simulink model "VTOLDynamics"  (R2024b)
settings: Solver=ode23t  StartTime=0.0  StopTime=10.0  FixedStep=0.001  RelTol=1e-3
undefined symbols (not defined in the file): const, contact, env, F, Flap_Activate, iniRoll, initPitch, iniYaw, Light, Limit, MIL, motorctrl, tiltIni, uavParam, uavParams, vIni, xGround, yGround, zGround
libraries: matrix_library x8, slpidlib x4, robotcorelib x4, aerolibasang x2, aerolibwind2 x2, sharedtransform x2, shared6dof x1, aerolibadyn x1, sharedutil x1, Uav_Electrical_lib x1, aerolibatmos2 x1
(part 1 of 3)
settings Model: DataDictionary=VTOLDynamicsData.sldd  Creator=The MathWorks, Inc.  LastModifiedBy=soung
settings DataIOCC: SaveOutput=off  SaveTime=off
settings GRTTargetCC: CombineOutputUpdateFcns=off  MatFileLogging=off

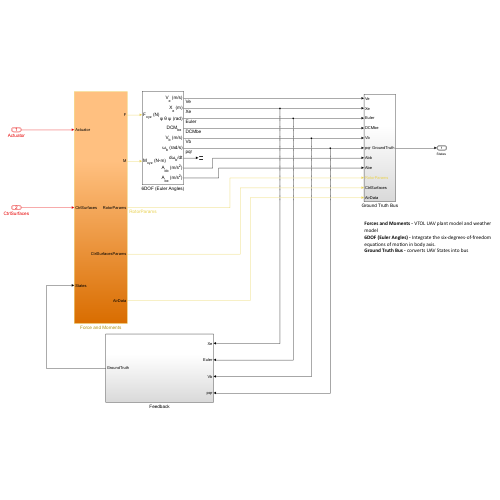
[thumbnail: Simulink's stored preview of the top-level diagram]
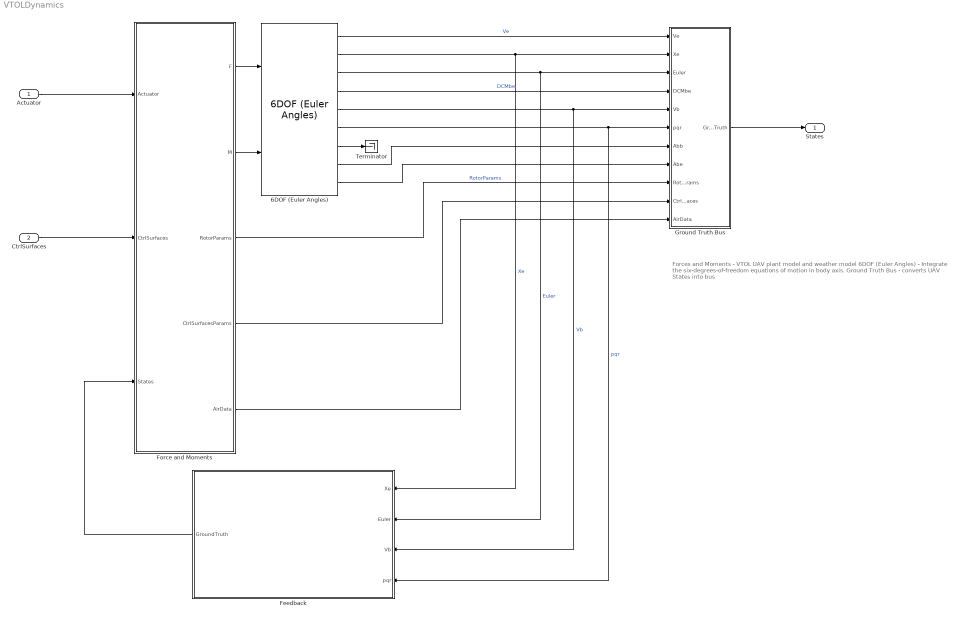
== system VTOLDynamics ==
  note: Forces and Moments - VTOL UAV plant model and weather model
      | 6DOF (Euler Angles) - Integrate the six-degrees-of-freedom equations of motion in body axis.
      | Ground Truth Bus - converts UAV States into bus
  Actuator : Inport  OutDataTypeStr=Bus: RotorCtrlBus  BusOutputAsStruct=on
  CtrlSurfaces : Inport  Port=2  OutDataTypeStr=Bus: FixedWingCtrlBus  BusOutputAsStruct=on
  6DOF (Euler Angles) : shared6dof/6DOF (Euler Angles)  units=Metric (MKS)  mtype=Fixed  rep=Euler Angles  xme_0=[xGround yGround zGround]  Vm_0=[vIni 0 0]  eul_0=[iniRoll initPitch iniYaw]  pm_0=[0 0 0]  mass_0=uavParams.geom.mass  mass_e=0.5  mass_f=2.0  inertia=[uavParams.geom.Ixx 0 0; 0 uavParams.geom.Iyy 0; 0 0 uavParams.geom.Izz]  inertia_e=eye(3)  inertia_f=2*eye(3)  k_quat=1.0  vre_flag=on  abi_flag=on  aMode=0  xme_statename=''  Vm_statename=''  eul_statename=''  quat_statename=''  pm_statename=''  mass_statename=''
  Feedback : Subsystem
  Force and Moments : Subsystem
  Ground Truth Bus : Subsystem
  Terminator : Terminator
  "States " : Outport  OutDataTypeStr=Bus: stateBus  BusOutputAsStruct=on
  wires:
  6DOF (Euler Angles)/4 -> Ground Truth Bus/4(DCMbe)  "DCMbe"
  Actuator/1 -> Force and Moments/1(Actuator)
  6DOF (Euler Angles)/2 -> Feedback/1(Xe), Ground Truth Bus/2(Xe)  "Xe"
  Force and Moments/5(AirData) -> Ground Truth Bus/11(AirData)
  6DOF (Euler Angles)/1 -> Ground Truth Bus/1(Ve)  "Ve"
  Force and Moments/3(RotorParams) -> Ground Truth Bus/9(RotorParams)  "RotorParams"
  6DOF (Euler Angles)/6 -> Ground Truth Bus/6(pqr), Feedback/4(pqr)  "pqr"
  CtrlSurfaces/1 -> Force and Moments/2(CtrlSurfaces)
  6DOF (Euler Angles)/7 -> Terminator/1
  6DOF (Euler Angles)/3 -> Feedback/2(Euler), Ground Truth Bus/3(Euler)  "Euler"
  6DOF (Euler Angles)/5 -> Ground Truth Bus/5(Vb), Feedback/3(Vb)  "Vb"
  Ground Truth Bus/1(GroundTruth) -> "States "/1
  6DOF (Euler Angles)/8 -> Ground Truth Bus/7(Abb)
  6DOF (Euler Angles)/9 -> Ground Truth Bus/8(Abe)
  Force and Moments/1(F) -> 6DOF (Euler Angles)/1
  Force and Moments/2(M) -> 6DOF (Euler Angles)/2
  Force and Moments/4(CtrlSurfacesParams) -> Ground Truth Bus/10(CtrlSurfaces)
  Feedback/1(GroundTruth) -> Force and Moments/3(States)

== system VTOLDynamics/Feedback ==
  Xe : Inport
  Euler : Inport  Port=2
  Vb : Inport  Port=3
  pqr : Inport  Port=4
  Reshape{,1..3} (4 alike) : Reshape  OutputDimensionality=Column vector (2-D)
  Bus Element Out3 : Outport  PortName=GroundTruth  Element=Xe
  Bus Element Out9 : Outport  PortName=GroundTruth  Element=pqr
  Bus Element Out6 : Outport  PortName=GroundTruth  Element=Vb
  Bus Element Out5 : Outport  PortName=GroundTruth  Element=Euler
  wires:
  Vb/1 -> Reshape/1
  Euler/1 -> Reshape1/1
  pqr/1 -> Reshape3/1
  Xe/1 -> Reshape2/1
  Reshape/1 -> Bus Element Out6/1
  Reshape1/1 -> Bus Element Out5/1
  Reshape2/1 -> Bus Element Out3/1
  Reshape3/1 -> Bus Element Out9/1

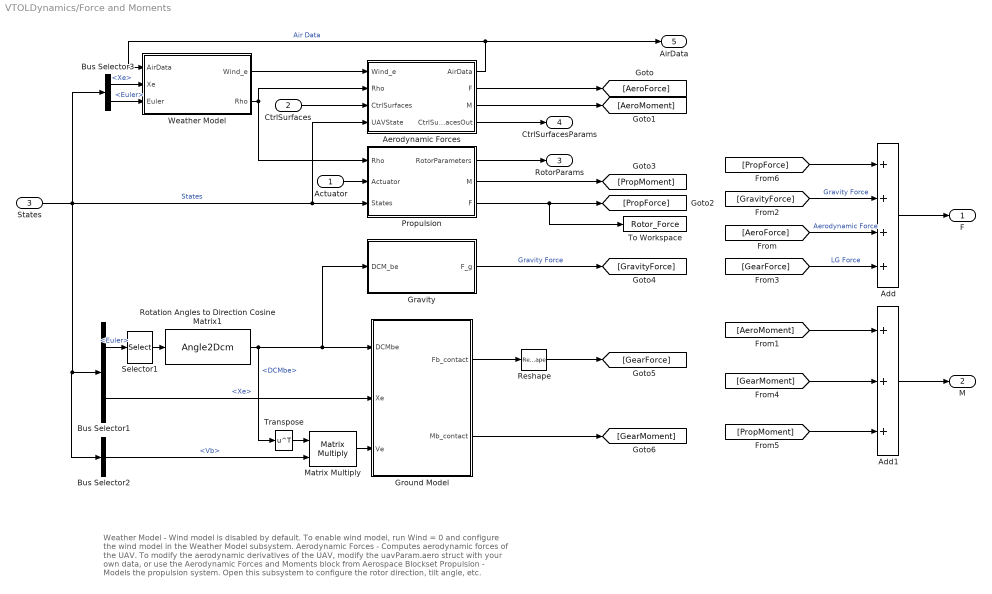
== system VTOLDynamics/Force and Moments ==
  note: Weather Model - Wind model is disabled by default. To enable wind model, run Wind = 0 and configure the wind model in the Weather Model subsystem.
      |
      | Aerodynamic Forces - Computes aerodynamic forces of the UAV. To modify the aerodynamic derivatives of the UAV, modify the uavParam.aero struct with your own data, or use the Aerodynamic Forces and Moments block from Aerospace Blockset
      |
      | Propulsion - Models the propulsion system. Open this subsystem to configure the rotor direction, tilt angle, etc.
  Actuator : Inport
  CtrlSurfaces : Inport  Port=2
  States : Inport  Port=3
  Add : Sum  Inputs=++++
  Add1 : Sum  Inputs=+++
  Aerodynamic Forces : Subsystem
  Bus Selector1 : BusSelector  OutputSignals=Euler,Xe
  Bus Selector2 : BusSelector  OutputSignals=Vb
  Bus Selector3 : BusSelector  OutputSignals=Xe,Euler
  Gravity : Subsystem
  Ground Model : Subsystem  VariantControl=Groundon==1
  Matrix Multiply : Product  Multiplication=Matrix(*)
  Propulsion : Subsystem
  Reshape : Reshape
  Rotation Angles to Direction Cosine Matrix1 : Angle2Dcm
      settings: AttributesFormatString=Rotation Order: %<rotationOrder>
  Selector1 : Selector  InputPortWidth=3  IndexOptions=Index vector (dialog)  Indices=[3 2 1]  OutputSizes=1
  To Workspace : ToWorkspace  VariableName=Rotor_Force  SaveFormat=Timeseries  SampleTime=-1
  Transpose : Math  Operator=transpose
  Weather Model : Subsystem  Variant=on  VariantControl=Weather Model
  F : Outport
  M : Outport  Port=2
  RotorParams : Outport  Port=3
  CtrlSurfacesParams : Outport  Port=4
  AirData : Outport  Port=5
  wires:
  [GravityForce] -> Add/2  "Gravity Force"
  Add/1 -> F/1
  CtrlSurfaces/1 -> Aerodynamic Forces/3(CtrlSurfaces)
  Add1/1 -> M/1
  [AeroForce] -> Add/3  "Aerodynamic Force"
  Aerodynamic Forces/2(F) -> [AeroForce]
  Actuator/1 -> Propulsion/2(Actuator)
  Propulsion/1(RotorParameters) -> RotorParams/1
  Aerodynamic Forces/1(AirData) -> Weather Model/1(AirData), AirData/1  "Air Data"
  Bus Selector3/1 -> Weather Model/2(Xe)  "<Xe>"
  Bus Selector3/2 -> Weather Model/3(Euler)  "<Euler>"
  Weather Model/1(Wind_e) -> Aerodynamic Forces/1(Wind_e)
  Weather Model/2(Rho) -> Propulsion/1(Rho), Aerodynamic Forces/2(Rho)
  Ground Model/1(Fb_contact) -> Reshape/1
  Aerodynamic Forces/3(M) -> [AeroMoment]
  Propulsion/3(F) -> To Workspace/1, [PropForce]
  Propulsion/2(M) -> [PropMoment]
  Gravity/1(F_g) -> [GravityForce]  "Gravity Force"
  Reshape/1 -> [GearForce]
  [GearForce] -> Add/4  "LG Force"
  Ground Model/2(Mb_contact) -> [GearMoment]
  [AeroMoment] -> Add1/1
  [GearMoment] -> Add1/2
  [PropMoment] -> Add1/3
  [PropForce] -> Add/1
  Aerodynamic Forces/4(CtrlSurfacesOut) -> CtrlSurfacesParams/1
  Bus Selector1/1 -> Selector1/1  "<Euler>"
  Bus Selector2/1 -> Matrix Multiply/2  "<Vb>"
  Rotation Angles to Direction Cosine Matrix1/1 -> Transpose/1, Gravity/1(DCM_be), Ground Model/1(DCMbe)  "<DCMbe>"
  Bus Selector1/2 -> Ground Model/2(Xe)  "<Xe>"
  Transpose/1 -> Matrix Multiply/1
  Selector1/1 -> Rotation Angles to Direction Cosine Matrix1/1
  States/1 -> Bus Selector2/1, Bus Selector1/1, Aerodynamic Forces/4(UAVState), Propulsion/3(States), Bus Selector3/1  "States"
  Matrix Multiply/1 -> Ground Model/3(Ve)

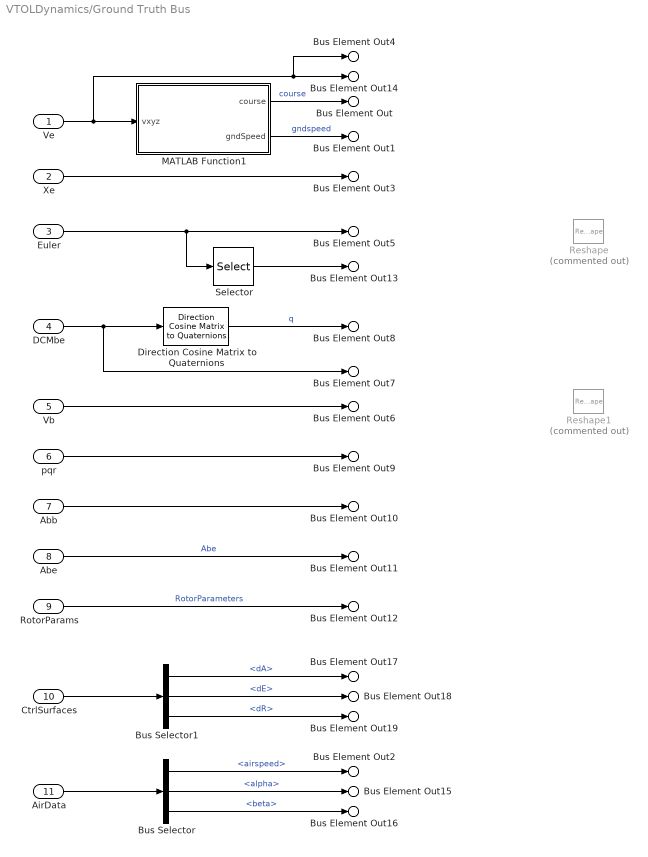
== system VTOLDynamics/Ground Truth Bus ==
  Ve : Inport
  Xe : Inport  Port=2
  Euler : Inport  Port=3
  DCMbe : Inport  Port=4
  Vb : Inport  Port=5
  pqr : Inport  Port=6
  Abb : Inport  Port=7
  Abe : Inport  Port=8
  RotorParams : Inport  Port=9
  CtrlSurfaces : Inport  Port=10
  AirData : Inport  Port=11
  Bus Selector : BusSelector  OutputSignals=airspeed,alpha,beta
  Bus Selector1 : BusSelector  OutputSignals=dA,dE,dR
  Direction Cosine Matrix to Quaternions : sharedtransform/Direction Cosine Matrix  to Quaternions  aMode=0  action=None  tolerance=eps(2)
      settings: LibrarySourceBlock=|
      | aerolibtransform2/Direction Cosine Matrix
      | to Quaternions
  MATLAB Function1 : MATLAB Function  TreatAsAtomicUnit=on
  Reshape : Reshape  Commented=on  OutputDimensionality=Column vector (2-D)
  Reshape1 : Reshape  Commented=on  OutputDimensionality=Row vector (2-D)
  Selector : Selector  InputPortWidth=3  IndexOptions=Index vector (dialog)  Indices=[3 2 1]  OutputSizes=1
  Bus Element Out : Outport  PortName=GroundTruth  Element=course
  Bus Element Out1 : Outport  PortName=GroundTruth  Element=gndspeed
  Bus Element Out2 : Outport  PortName=GroundTruth  Element=airspeed
  Bus Element Out3 : Outport  PortName=GroundTruth  Element=Xe
  Bus Element Out4 : Outport  PortName=GroundTruth  Element=Ve
  Bus Element Out7 : Outport  PortName=GroundTruth  Element=DCMbe
  Bus Element Out8 : Outport  PortName=GroundTruth  Element=q
  Bus Element Out9 : Outport  PortName=GroundTruth  Element=pqr
  Bus Element Out6 : Outport  PortName=GroundTruth  Element=Vb
  Bus Element Out10 : Outport  PortName=GroundTruth  Element=Abb
  Bus Element Out11 : Outport  PortName=GroundTruth  Element=Abe
  Bus Element Out5 : Outport  PortName=GroundTruth  Element=Euler
  Bus Element Out12 : Outport  PortName=GroundTruth  Element=RotorParameters
  Bus Element Out13 : Outport  PortName=GroundTruth  Element=ypr
  Bus Element Out14 : Outport  PortName=GroundTruth  Element=Ve_ground
  Bus Element Out15 : Outport  PortName=GroundTruth  Element=aoa
  Bus Element Out16 : Outport  PortName=GroundTruth  Element=aos
  Bus Element Out17 : Outport  PortName=GroundTruth  Element=aileron
  Bus Element Out18 : Outport  PortName=GroundTruth  Element=elevator
  Bus Element Out19 : Outport  PortName=GroundTruth  Element=rudder
  wires:
  DCMbe/1 -> Bus Element Out7/1, Direction Cosine Matrix to Quaternions/1
  Ve/1 -> Bus Element Out14/1, Bus Element Out4/1, MATLAB Function1/1(vxyz)
  MATLAB Function1/1(course) -> Bus Element Out/1  "course"
  MATLAB Function1/2(gndSpeed) -> Bus Element Out1/1  "gndspeed"
  Direction Cosine Matrix to Quaternions/1 -> Bus Element Out8/1  "q"
  pqr/1 -> Bus Element Out9/1
  Abb/1 -> Bus Element Out10/1
  Abe/1 -> Bus Element Out11/1  "Abe"
  RotorParams/1 -> Bus Element Out12/1  "RotorParameters"
  Selector/1 -> Bus Element Out13/1
  Euler/1 -> Selector/1, Bus Element Out5/1
  Vb/1 -> Bus Element Out6/1
  Xe/1 -> Bus Element Out3/1
  AirData/1 -> Bus Selector/1
  Bus Selector/1 -> Bus Element Out2/1  "<airspeed>"
  Bus Selector/2 -> Bus Element Out15/1  "<alpha>"
  Bus Selector/3 -> Bus Element Out16/1  "<beta>"
  CtrlSurfaces/1 -> Bus Selector1/1
  Bus Selector1/1 -> Bus Element Out17/1  "<dA>"
  Bus Selector1/2 -> Bus Element Out18/1  "<dE>"
  Bus Selector1/3 -> Bus Element Out19/1  "<dR>"

== system VTOLDynamics/Force and Moments/Aerodynamic Forces ==
  Wind_e : Inport
  Rho : Inport  Port=2
  CtrlSurfaces : Inport  Port=3
  UAVState : Inport  Port=4
  Bus Selector2 : BusSelector  OutputSignals=Euler,Vb,pqr,Xe
  Compute Air Data : Subsystem  TreatAsAtomicUnit=on  VariantControl=use_aerospace_blocks == 1
  Compute Body Frame Forces and Moments : Subsystem
  Matrix Multiply : Product  Multiplication=Matrix(*)
  Matrix Multiply1 : Product  Multiplication=Matrix(*)
  Rotation Angles to Direction Cosine Matrix1 : Angle2Dcm
      settings: AttributesFormatString=Rotation Order: %<rotationOrder>
  Selector1 : Selector  InputPortWidth=3  IndexOptions=Index vector (dialog)  Indices=[3 2 1]  OutputSizes=1
  Transpose : Math  Operator=transpose
  Vair : Sum  Inputs=+-  InputSameDT=on  SaturateOnIntegerOverflow=on  OutDataTypeStr=Inherit: Same as first input
  AirData : Outport  VectorParamsAs1DForOutWhenUnconnected=off
  F : Outport  Port=2
  M : Outport  Port=3
  CtrlSurfacesOut : Outport  Port=4
  wires:
  Compute Body Frame Forces and Moments/1(F_b) -> F/1
  CtrlSurfaces/1 -> Compute Body Frame Forces and Moments/2(CtrlSurfaces)
  Compute Air Data/1(AirData) -> Compute Body Frame Forces and Moments/1(AirData), AirData/1
  Compute Body Frame Forces and Moments/2(M_b) -> M/1
  Matrix Multiply/1 -> Compute Body Frame Forces and Moments/3(Vb), Compute Air Data/1(Vb)
  Rho/1 -> Compute Air Data/2(Rho)
  Vair/1 -> Matrix Multiply/2
  Wind_e/1 -> Vair/2
  Compute Body Frame Forces and Moments/3(CtrlSurfacesStates) -> CtrlSurfacesOut/1
  Bus Selector2/3 -> Compute Body Frame Forces and Moments/4(p,q,r)  "<pqr>"
  UAVState/1 -> Bus Selector2/1
  Matrix Multiply1/1 -> Vair/1
  Rotation Angles to Direction Cosine Matrix1/1 -> Matrix Multiply/1, Transpose/1  "<DCMbe>"
  Selector1/1 -> Rotation Angles to Direction Cosine Matrix1/1
  Transpose/1 -> Matrix Multiply1/1
  Bus Selector2/2 -> Matrix Multiply1/2  "<Vb>"
  Bus Selector2/1 -> Selector1/1  "<Euler>"
  Bus Selector2/4 -> Compute Body Frame Forces and Moments/5(Xe)  "<Xe>"

== system VTOLDynamics/Force and Moments/Gravity ==
  DCM_be : Inport
  Constant : Constant  Value=[0 0 const.g]'
  Gain : Gain  Gain=uavParams.geom.mass
  Matrix Multiply : Product  Multiplication=Matrix(*)
  F_g : Outport
  wires:
  Matrix Multiply/1 -> Gain/1
  Constant/1 -> Matrix Multiply/2
  DCM_be/1 -> Matrix Multiply/1
  Gain/1 -> F_g/1

== system VTOLDynamics/Force and Moments/Ground Model ==
  note: Body is assumed to be a rigid point mass on ground for contact force calculations.
      |
      | Normal force is modelled as a spring mass damper.
      |
      | Friction is modelled using Soft Coulomb model.
  note: #4, 25/05/20, MH, Not Fixed
      | Moment created by the landing gear is set to be
      | zero, which causes simulator divergence
      | Can be fixed by updating the tri-cycle landing
      | gear model
  DCMbe : Inport
  Xe : Inport  Port=2
  Ve : Inport  Port=3
  Constant : Constant  Value=[0 0 0]  SampleTime=-1
  Friction Force : Subsystem
  Matrix Multiply : Product  Multiplication=Matrix(*)
  Mux1 : Mux  Inputs=2
  Normal Force : Subsystem
  Selector : Selector  InputPortWidth=3  IndexOptions=Index vector (dialog)  Indices=[3]  OutputSizes=1
  Selector1 : Selector  InputPortWidth=3  IndexOptions=Index vector (dialog)  Indices=[3]  OutputSizes=1
  Selector2 : Selector  InputPortWidth=3  IndexOptions=Index vector (dialog)  Indices=[1,2]  OutputSizes=1
  Unary Minus1 : UnaryMinus
  Fb_contact : Outport
  Mb_contact : Outport  Port=2
  wires:
  Xe/1 -> Selector/1
  Ve/1 -> Selector2/1, Selector1/1
  Selector1/1 -> Normal Force/1(Vz)
  Selector/1 -> Normal Force/2(Z)
  DCMbe/1 -> Matrix Multiply/1
  Normal Force/1(Normal) -> Friction Force/2(Fn), Unary Minus1/1
  Unary Minus1/1 -> Mux1/2
  Selector2/1 -> Friction Force/1(V)
  Friction Force/1(Friction) -> Mux1/1
  Constant/1 -> Mb_contact/1
  Mux1/1 -> Matrix Multiply/2
  Matrix Multiply/1 -> Fb_contact/1

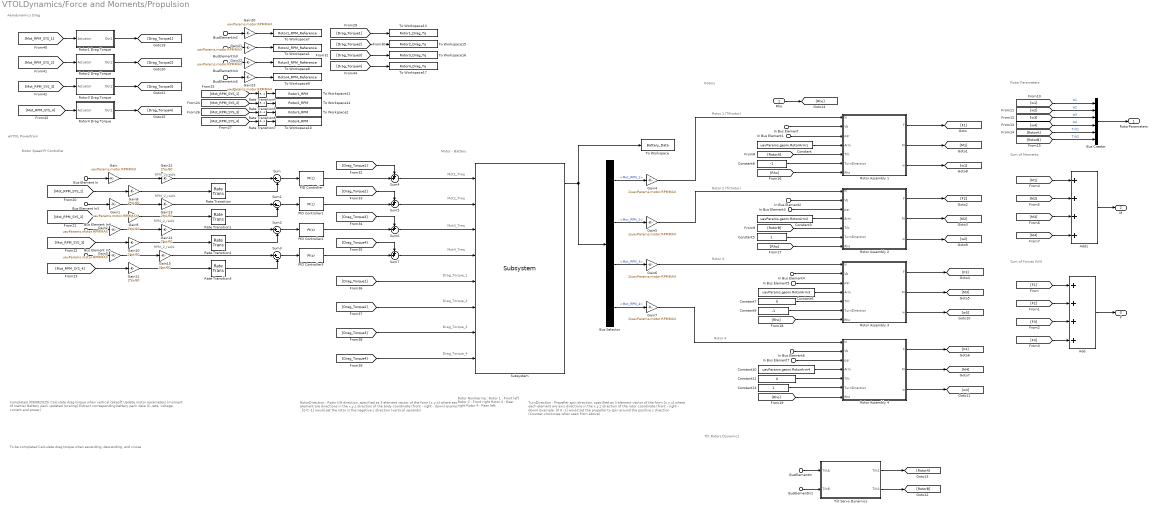
== system VTOLDynamics/Force and Moments/Propulsion ==
  note: RPM_2_rad/s
  note: Motor - Battery
  note: TurnDirection : Propeller spin direction, specified as 3 element vector of the form [x y z] where each element are axis directions in the x,y,z direction of the rotor coordinate (front - right - down)
      |
      | Example: [0 0 -1] would set the propeller to spin around the positive z direction (Counter-clockwise when seen from above)
  note: RotorDirection : Rotor tilt direction, specified as 3 element vector of the form [x y z] where each element are directions in the x,y,z direction of the body coordinate (front - right - down)
      |
      | example : [0 0 -1] would set the rotor in the negative z direction (vertical upwards)
  note: Rotor Numbering :
      | Rotor 1 : Front left
      | Rotor 2 : Front right
      | Rotor 3 : Rear right
      | Rotor 4 : Rear left
  note: Sum of Moments
  note: Rotor 1 (Tiltrotor)
  note: eVTOL Powertrain
  note: Rotor 2 (Titlrotor)
  note: Rotor 3
  note: Rotor 4
  note: Sum of Forces (kN)
  note: Rotor Parameters
  note: Rotors
  note: Motor Speed PI Controller
  note: RPM_2_rad/s
  note: RPM_2_rad/s
  note: RPM_2_rad/s
  note: Mot1_Treq
  note: Mot2_Treq
  note: Mot3_Treq
  note: Mot4_Treq
  note: Completed (09/08/2025)
      |
      | Calculate drag torque when vertical takeoff
      | Update motor parameters (moment of inertia)
      | Battery pack updated (scaling)
      | Extract corresponding battery pack data (C-rate, voltage, current and power)
  note: Aerodynamics Drag
  note: Drag_Torque_1
  note: Drag_Torque_2
  note: Drag_Torque_3
  note: Drag_Torque_4
  note: Tilt Rotors Dynamics
  note: To be completed
      |
      | Calculate drag torque when ascending, descending, and cruise
  Rho : Inport
  Bus Element In : Inport  Port=2  PortName=Actuator  Element=w1
  BusElementIn2 : Inport  Port=2  PortName=Actuator  Element=w1
  Bus Element In3 : Inport  Port=2  PortName=Actuator  Element=w2
  BusElementIn3 : Inport  Port=2  PortName=Actuator  Element=w2
  Bus Element In5 : Inport  Port=2  PortName=Actuator  Element=w4
  BusElementIn5 : Inport  Port=2  PortName=Actuator  Element=w4
  Bus Element In4 : Inport  Port=2  PortName=Actuator  Element=w3
  BusElementIn4 : Inport  Port=2  PortName=Actuator  Element=w3
  BusElementIn : Inport  Port=2  PortName=Actuator  Element=Tilt1
  BusElementIn1 : Inport  Port=2  PortName=Actuator  Element=Tilt2
  In Bus Element{,2,4,6} (4 alike) : Inport  Port=3  PortName=States  Element=Vb
  In Bus Element{1,3,5,7} (4 alike) : Inport  Port=3  PortName=States  Element=pqr
  Add : Sum  Inputs=++++
  Add1 : Sum  Inputs=++++
  Bus Creator : BusCreator  Inputs=6  OutDataTypeStr=Bus: RotorCtrlBus
  Bus Selector : BusSelector  OutputSignals=Mot_RPM_1,Mot_RPM_2,Mot_RPM_3,Mot_RPM_4
  Constant : Constant  Value=uavParams.geom.RotorArm1
  Constant10 : Constant  Value=uavParams.geom.RotorArm4
  Constant11 : Constant  Value=0
  Constant13 : Constant
  Constant3 : Constant  Value=uavParams.geom.RotorArm2
  Constant5 : Constant
  Constant6 : Constant  Value=uavParams.geom.RotorArm3
  Constant7 : Constant  Value=0
  Constant8 : Constant  Value=-1
  Constant9 : Constant  Value=-1
  Gain{,1..3,20..23} (8 alike) : Gain  Gain=uavParams.motor.RPMMAX
  Gain{8..15} (8 alike) : Gain  Gain=2*pi/60
  Gain{4..7} (4 alike) : Gain  Gain=1/uavParams.motor.RPMMAX
  PID Controller : slpidlib/PID Controller  Controller=PI  Form=Parallel  TimeDomain=Discrete-time  UseExternalTs=off  SampleTime=0.005  IntegratorMethod=Forward Euler  FilterMethod=Forward Euler  ControllerParametersSource=internal  P=motorctrl.p  I=motorctrl.i  UseKiTs=off  D=motorctrl.d  UseExternalDerivativeSource=off  N=motorctrl.n  UseFilter=on  TunerSelectOption=Transfer Function Based (PID Tuner App)  InitialConditionSource=internal  InitialConditionForIntegrator=0  InitialConditionForFilter=0  DifferentiatorICPrevScaledInput=0  ExternalReset=none  TrackingMode=off  Kt=1  LimitOutput=on  SatLimitsSource=internal  UpperSaturationLimit=Limit  LowerSaturationLimit=-Limit  LinearizeAsGain=on  AntiWindupMode=none  Kb=1  LimitIntegrator=off  UpperIntegratorSaturationLimit=inf  LowerIntegratorSaturationLimit=-inf  POutMin=[]  POutMax=[]  IOutMin=[]  IOutMax=[]  DOutMin=[]  DOutMax=[]  NOutMin=[]  NOutMax=[]  SumOutMin=[]  SumOutMax=[]  SaturationOutMin=[]  SaturationOutMax=[]  PParamMin=[]  PParamMax=[]  IParamMin=[]  IParamMax=[]  DParamMin=[]  DParamMax=[]  NParamMin=[]  NParamMax=[]  KbParamMin=[]  KbParamMax=[]  KtParamMin=[]  KtParamMax=[]  KbOutMin=[]  KbOutMax=[]  KtOutMin=[]  KtOutMax=[]  IntegratorOutMin=[]  IntegratorOutMax=[]  FilterOutMin=[]  FilterOutMax=[]  SumI1OutMin=[]  SumI1OutMax=[]  SumI2OutMin=[]  SumI2OutMax=[]  SumI3OutMin=[]  SumI3OutMax=[]  SumI4OutMin=[]  SumI4OutMax=[]  SumDOutMin=[]  SumDOutMax=[]  DifferentiatorOutMin=[]  DifferentiatorOutMax=[]  FilterDiffOutCoefMin=[]  FilterDiffOutCoefMax=[]  ReciprocalOutMin=[]  ReciprocalOutMax=[]  SumDenOutMin=[]  SumDenOutMax=[]  SumNumOutMin=[]  SumNumOutMax=[]  DivideOutMin=[]  DivideOutMax=[]  UdiffTsProdOutMin=[]  UdiffTsProdOutMax=[]  NTsProdOutMin=[]  NTsProdOutMax=[]  UintegralTsProdOutMin=[]  UintegralTsProdOutMax=[]  UngainTsProdOutMin=[]  UngainTsProdOutMax=[]  ClampingZeroOutDataTypeStr=Inherit: Inherit via back propagation  ClampingZeroOutMin=[]  ClampingZeroOutMax=[]  FilterDenConstantOutDataTypeStr=Inherit: Inherit via back propagation  FilterDenConstantOutMin=[]  FilterDenConstantOutMax=[]  PCopyOutDataTypeStr=Inherit: Inherit via back propagation  PCopyOutMin=[]  PCopyOutMax=[]  NCopyOutDataTypeStr=Inherit: Inherit via back propagation  NCopyOutMin=[]  NCopyOutMax=[]  IntegratorContinuousStateAttributes=''  IntegratorStateMustResolveToSignalObject=off  IntegratorRTWStateStorageClass=Auto  FilterContinuousStateAttributes=''  FilterStateMustResolveToSignalObject=off  FilterRTWStateStorageClass=Auto  ParallelPVariant=InternalParameters  IdealPVariant=Disabled  IVariant=InternalParameters  DVariant=Disabled  IntegratorVariant=Discrete  SatVariant=Enabled  AWVariant=Passthrough  PCopyVariant=Disabled  TRVariant=Disabled  FdbkBlocksVariant=Forward  IdealPFdbkVariant=Disabled  SatFdbkVariant=Disabled  DerivativeFilterVariant=Disabled  NVariant=Disabled  NCopyVariant=Disabled_SignalSpec  FilterICVariant=Disabled  IntegratorICVariant=InternalICs  ExternalResetVariant=Disabled  TRSumVariant=Passthrough  SumFdbkVariant=Disabled  SumVariant=Sum_PI  TsampFilterVariant=InternalTs  TsampNgainVariant=Passthrough  TsampIntegralVariant=Disabled_SignalSpec  ExternalSaturationOutDataTypeStr=Inherit: Same as second input  DerivativeSourceVariant=Disabled  PreIntVariant=InternalPreInt
  PID Controller1 : slpidlib/PID Controller  Controller=PI  Form=Parallel  TimeDomain=Discrete-time  UseExternalTs=off  SampleTime=0.005  IntegratorMethod=Forward Euler  FilterMethod=Forward Euler  ControllerParametersSource=internal  P=motorctrl.p  I=motorctrl.i  UseKiTs=off  D=motorctrl.d  UseExternalDerivativeSource=off  N=motorctrl.n  UseFilter=on  TunerSelectOption=Transfer Function Based (PID Tuner App)  InitialConditionSource=internal  InitialConditionForIntegrator=0  InitialConditionForFilter=0  DifferentiatorICPrevScaledInput=0  ExternalReset=none  TrackingMode=off  Kt=1  LimitOutput=on  SatLimitsSource=internal  UpperSaturationLimit=Limit  LowerSaturationLimit=-Limit  LinearizeAsGain=on  AntiWindupMode=none  Kb=1  LimitIntegrator=off  UpperIntegratorSaturationLimit=inf  LowerIntegratorSaturationLimit=-inf  POutMin=[]  POutMax=[]  IOutMin=[]  IOutMax=[]  DOutMin=[]  DOutMax=[]  NOutMin=[]  NOutMax=[]  SumOutMin=[]  SumOutMax=[]  SaturationOutMin=[]  SaturationOutMax=[]  PParamMin=[]  PParamMax=[]  IParamMin=[]  IParamMax=[]  DParamMin=[]  DParamMax=[]  NParamMin=[]  NParamMax=[]  KbParamMin=[]  KbParamMax=[]  KtParamMin=[]  KtParamMax=[]  KbOutMin=[]  KbOutMax=[]  KtOutMin=[]  KtOutMax=[]  IntegratorOutMin=[]  IntegratorOutMax=[]  FilterOutMin=[]  FilterOutMax=[]  SumI1OutMin=[]  SumI1OutMax=[]  SumI2OutMin=[]  SumI2OutMax=[]  SumI3OutMin=[]  SumI3OutMax=[]  SumI4OutMin=[]  SumI4OutMax=[]  SumDOutMin=[]  SumDOutMax=[]  DifferentiatorOutMin=[]  DifferentiatorOutMax=[]  FilterDiffOutCoefMin=[]  FilterDiffOutCoefMax=[]  ReciprocalOutMin=[]  ReciprocalOutMax=[]  SumDenOutMin=[]  SumDenOutMax=[]  SumNumOutMin=[]  SumNumOutMax=[]  DivideOutMin=[]  DivideOutMax=[]  UdiffTsProdOutMin=[]  UdiffTsProdOutMax=[]  NTsProdOutMin=[]  NTsProdOutMax=[]  UintegralTsProdOutMin=[]  UintegralTsProdOutMax=[]  UngainTsProdOutMin=[]  UngainTsProdOutMax=[]  ClampingZeroOutDataTypeStr=Inherit: Inherit via back propagation  ClampingZeroOutMin=[]  ClampingZeroOutMax=[]  FilterDenConstantOutDataTypeStr=Inherit: Inherit via back propagation  FilterDenConstantOutMin=[]  FilterDenConstantOutMax=[]  PCopyOutDataTypeStr=Inherit: Inherit via back propagation  PCopyOutMin=[]  PCopyOutMax=[]  NCopyOutDataTypeStr=Inherit: Inherit via back propagation  NCopyOutMin=[]  NCopyOutMax=[]  IntegratorContinuousStateAttributes=''  IntegratorStateMustResolveToSignalObject=off  IntegratorRTWStateStorageClass=Auto  FilterContinuousStateAttributes=''  FilterStateMustResolveToSignalObject=off  FilterRTWStateStorageClass=Auto  ParallelPVariant=InternalParameters  IdealPVariant=Disabled  IVariant=InternalParameters  DVariant=Disabled  IntegratorVariant=Discrete  SatVariant=Enabled  AWVariant=Passthrough  PCopyVariant=Disabled  TRVariant=Disabled  FdbkBlocksVariant=Forward  IdealPFdbkVariant=Disabled  SatFdbkVariant=Disabled  DerivativeFilterVariant=Disabled  NVariant=Disabled  NCopyVariant=Disabled_SignalSpec  FilterICVariant=Disabled  IntegratorICVariant=InternalICs  ExternalResetVariant=Disabled  TRSumVariant=Passthrough  SumFdbkVariant=Disabled  SumVariant=Sum_PI  TsampFilterVariant=InternalTs  TsampNgainVariant=Passthrough  TsampIntegralVariant=Disabled_SignalSpec  ExternalSaturationOutDataTypeStr=Inherit: Same as second input  DerivativeSourceVariant=Disabled  PreIntVariant=InternalPreInt
  PID Controller2 : slpidlib/PID Controller  Controller=PI  Form=Parallel  TimeDomain=Discrete-time  UseExternalTs=off  SampleTime=0.005  IntegratorMethod=Forward Euler  FilterMethod=Forward Euler  ControllerParametersSource=internal  P=motorctrl.p  I=motorctrl.i  UseKiTs=off  D=motorctrl.d  UseExternalDerivativeSource=off  N=motorctrl.n  UseFilter=on  TunerSelectOption=Transfer Function Based (PID Tuner App)  InitialConditionSource=internal  InitialConditionForIntegrator=0  InitialConditionForFilter=0  DifferentiatorICPrevScaledInput=0  ExternalReset=none  TrackingMode=off  Kt=1  LimitOutput=on  SatLimitsSource=internal  UpperSaturationLimit=Limit  LowerSaturationLimit=-Limit  LinearizeAsGain=on  AntiWindupMode=none  Kb=1  LimitIntegrator=off  UpperIntegratorSaturationLimit=inf  LowerIntegratorSaturationLimit=-inf  POutMin=[]  POutMax=[]  IOutMin=[]  IOutMax=[]  DOutMin=[]  DOutMax=[]  NOutMin=[]  NOutMax=[]  SumOutMin=[]  SumOutMax=[]  SaturationOutMin=[]  SaturationOutMax=[]  PParamMin=[]  PParamMax=[]  IParamMin=[]  IParamMax=[]  DParamMin=[]  DParamMax=[]  NParamMin=[]  NParamMax=[]  KbParamMin=[]  KbParamMax=[]  KtParamMin=[]  KtParamMax=[]  KbOutMin=[]  KbOutMax=[]  KtOutMin=[]  KtOutMax=[]  IntegratorOutMin=[]  IntegratorOutMax=[]  FilterOutMin=[]  FilterOutMax=[]  SumI1OutMin=[]  SumI1OutMax=[]  SumI2OutMin=[]  SumI2OutMax=[]  SumI3OutMin=[]  SumI3OutMax=[]  SumI4OutMin=[]  SumI4OutMax=[]  SumDOutMin=[]  SumDOutMax=[]  DifferentiatorOutMin=[]  DifferentiatorOutMax=[]  FilterDiffOutCoefMin=[]  FilterDiffOutCoefMax=[]  ReciprocalOutMin=[]  ReciprocalOutMax=[]  SumDenOutMin=[]  SumDenOutMax=[]  SumNumOutMin=[]  SumNumOutMax=[]  DivideOutMin=[]  DivideOutMax=[]  UdiffTsProdOutMin=[]  UdiffTsProdOutMax=[]  NTsProdOutMin=[]  NTsProdOutMax=[]  UintegralTsProdOutMin=[]  UintegralTsProdOutMax=[]  UngainTsProdOutMin=[]  UngainTsProdOutMax=[]  ClampingZeroOutDataTypeStr=Inherit: Inherit via back propagation  ClampingZeroOutMin=[]  ClampingZeroOutMax=[]  FilterDenConstantOutDataTypeStr=Inherit: Inherit via back propagation  FilterDenConstantOutMin=[]  FilterDenConstantOutMax=[]  PCopyOutDataTypeStr=Inherit: Inherit via back propagation  PCopyOutMin=[]  PCopyOutMax=[]  NCopyOutDataTypeStr=Inherit: Inherit via back propagation  NCopyOutMin=[]  NCopyOutMax=[]  IntegratorContinuousStateAttributes=''  IntegratorStateMustResolveToSignalObject=off  IntegratorRTWStateStorageClass=Auto  FilterContinuousStateAttributes=''  FilterStateMustResolveToSignalObject=off  FilterRTWStateStorageClass=Auto  ParallelPVariant=InternalParameters  IdealPVariant=Disabled  IVariant=InternalParameters  DVariant=Disabled  IntegratorVariant=Discrete  SatVariant=Enabled  AWVariant=Passthrough  PCopyVariant=Disabled  TRVariant=Disabled  FdbkBlocksVariant=Forward  IdealPFdbkVariant=Disabled  SatFdbkVariant=Disabled  DerivativeFilterVariant=Disabled  NVariant=Disabled  NCopyVariant=Disabled_SignalSpec  FilterICVariant=Disabled  IntegratorICVariant=InternalICs  ExternalResetVariant=Disabled  TRSumVariant=Passthrough  SumFdbkVariant=Disabled  SumVariant=Sum_PI  TsampFilterVariant=InternalTs  TsampNgainVariant=Passthrough  TsampIntegralVariant=Disabled_SignalSpec  ExternalSaturationOutDataTypeStr=Inherit: Same as second input  DerivativeSourceVariant=Disabled  PreIntVariant=InternalPreInt
  PID Controller3 : slpidlib/PID Controller  Controller=PI  Form=Parallel  TimeDomain=Discrete-time  UseExternalTs=off  SampleTime=0.005  IntegratorMethod=Forward Euler  FilterMethod=Forward Euler  ControllerParametersSource=internal  P=motorctrl.p  I=motorctrl.i  UseKiTs=off  D=motorctrl.d  UseExternalDerivativeSource=off  N=motorctrl.n  UseFilter=on  TunerSelectOption=Transfer Function Based (PID Tuner App)  InitialConditionSource=internal  InitialConditionForIntegrator=0  InitialConditionForFilter=0  DifferentiatorICPrevScaledInput=0  ExternalReset=none  TrackingMode=off  Kt=1  LimitOutput=on  SatLimitsSource=internal  UpperSaturationLimit=Limit  LowerSaturationLimit=-Limit  LinearizeAsGain=off  AntiWindupMode=none  Kb=1  LimitIntegrator=off  UpperIntegratorSaturationLimit=inf  LowerIntegratorSaturationLimit=-inf  POutMin=[]  POutMax=[]  IOutMin=[]  IOutMax=[]  DOutMin=[]  DOutMax=[]  NOutMin=[]  NOutMax=[]  SumOutMin=[]  SumOutMax=[]  SaturationOutMin=[]  SaturationOutMax=[]  PParamMin=[]  PParamMax=[]  IParamMin=[]  IParamMax=[]  DParamMin=[]  DParamMax=[]  NParamMin=[]  NParamMax=[]  KbParamMin=[]  KbParamMax=[]  KtParamMin=[]  KtParamMax=[]  KbOutMin=[]  KbOutMax=[]  KtOutMin=[]  KtOutMax=[]  IntegratorOutMin=[]  IntegratorOutMax=[]  FilterOutMin=[]  FilterOutMax=[]  SumI1OutMin=[]  SumI1OutMax=[]  SumI2OutMin=[]  SumI2OutMax=[]  SumI3OutMin=[]  SumI3OutMax=[]  SumI4OutMin=[]  SumI4OutMax=[]  SumDOutMin=[]  SumDOutMax=[]  DifferentiatorOutMin=[]  DifferentiatorOutMax=[]  FilterDiffOutCoefMin=[]  FilterDiffOutCoefMax=[]  ReciprocalOutMin=[]  ReciprocalOutMax=[]  SumDenOutMin=[]  SumDenOutMax=[]  SumNumOutMin=[]  SumNumOutMax=[]  DivideOutMin=[]  DivideOutMax=[]  UdiffTsProdOutMin=[]  UdiffTsProdOutMax=[]  NTsProdOutMin=[]  NTsProdOutMax=[]  UintegralTsProdOutMin=[]  UintegralTsProdOutMax=[]  UngainTsProdOutMin=[]  UngainTsProdOutMax=[]  ClampingZeroOutDataTypeStr=Inherit: Inherit via back propagation  ClampingZeroOutMin=[]  ClampingZeroOutMax=[]  FilterDenConstantOutDataTypeStr=Inherit: Inherit via back propagation  FilterDenConstantOutMin=[]  FilterDenConstantOutMax=[]  PCopyOutDataTypeStr=Inherit: Inherit via back propagation  PCopyOutMin=[]  PCopyOutMax=[]  NCopyOutDataTypeStr=Inherit: Inherit via back propagation  NCopyOutMin=[]  NCopyOutMax=[]  IntegratorContinuousStateAttributes=''  IntegratorStateMustResolveToSignalObject=off  IntegratorRTWStateStorageClass=Auto  FilterContinuousStateAttributes=''  FilterStateMustResolveToSignalObject=off  FilterRTWStateStorageClass=Auto  ParallelPVariant=InternalParameters  IdealPVariant=Disabled  IVariant=InternalParameters  DVariant=Disabled  IntegratorVariant=Discrete  SatVariant=Enabled  AWVariant=Passthrough  PCopyVariant=Disabled  TRVariant=Disabled  FdbkBlocksVariant=Forward  IdealPFdbkVariant=Disabled  SatFdbkVariant=Disabled  DerivativeFilterVariant=Disabled  NVariant=Disabled  NCopyVariant=Disabled_SignalSpec  FilterICVariant=Disabled  IntegratorICVariant=InternalICs  ExternalResetVariant=Disabled  TRSumVariant=Passthrough  SumFdbkVariant=Disabled  SumVariant=Sum_PI  TsampFilterVariant=InternalTs  TsampNgainVariant=Passthrough  TsampIntegralVariant=Disabled_SignalSpec  ExternalSaturationOutDataTypeStr=Inherit: Same as second input  DerivativeSourceVariant=Disabled  PreIntVariant=InternalPreInt
  Rate Transition{,1..7} (8 alike) : RateTransition
  Rotor Assembly 1 : Subsystem
  Rotor Assembly 2 : Subsystem
  Rotor Assembly 3 : Subsystem
  Rotor Assembly 4 : Subsystem
  Rotor1 Drag Torque : Subsystem
  Rotor2 Drag Torque : Subsystem
  Rotor3 Drag Torque : Subsystem
  Rotor4 Drag Torque : Subsystem
  Subsystem : Uav_Electrical_lib/Subsystem  SystemSampleTime=-1  VariantActivationTime=update diagram  AllowFlexibleInterface=on  Latency=0  AutoFrameSizeCalculation=off
      link override System Level/Bus Selector: OutputSignals=Drag1_Tq_Nm,Drag2_Tq_Nm,Drag3_Tq_Nm,Drag4_Tq_Nm
      mask Display: image('Snipaste_2025-07-29_12-40-51.jpg');
  Sum{,1..3} (4 alike) : Sum  Inputs=|+-
  Sum{4..7} (4 alike) : Sum  Inputs=++|
  Tilt Servo Dynamics : Subsystem
  To Workspace : ToWorkspace  VariableName=Battery_Data  SaveFormat=Timeseries  SampleTime=-1
  To Workspace1 : ToWorkspace  VariableName=Rotor2_RPM_Reference  SaveFormat=Timeseries  SampleTime=-1
  To Workspace10 : ToWorkspace  VariableName=Rotor4_RPM  SaveFormat=Timeseries  SampleTime=-1
  To Workspace11 : ToWorkspace  VariableName=Rotor1_RPM  SaveFormat=Timeseries  SampleTime=-1
  To Workspace13 : ToWorkspace  VariableName=Rotor1_Drag_Tq  SaveFormat=Timeseries  SampleTime=-1
  To Workspace14 : ToWorkspace  VariableName=Rotor2_RPM  SaveFormat=Timeseries  SampleTime=-1
  To Workspace15 : ToWorkspace  VariableName=Rotor2_Drag_Tq  SaveFormat=Timeseries  SampleTime=-1
  To Workspace16 : ToWorkspace  VariableName=Rotor3_Drag_Tq  SaveFormat=Timeseries  SampleTime=-1
  To Workspace17 : ToWorkspace  VariableName=Rotor4_Drag_Tq  SaveFormat=Timeseries  SampleTime=-1
  To Workspace2 : ToWorkspace  VariableName=Rotor3_RPM  SaveFormat=Timeseries  SampleTime=-1
  To Workspace7 : ToWorkspace  VariableName=Rotor1_RPM_Reference  SaveFormat=Timeseries  SampleTime=-1
  To Workspace8 : ToWorkspace  VariableName=Rotor3_RPM_Reference  SaveFormat=Timeseries  SampleTime=-1
  To Workspace9 : ToWorkspace  VariableName=Rotor4_RPM_Reference  SaveFormat=Timeseries  SampleTime=-1
  RotorParameters : Outport
  M : Outport  Port=2
  F : Outport  Port=3
  wires:
  In Bus Element/1 -> Rotor Assembly 1/2(Vb)
  In Bus Element1/1 -> Rotor Assembly 1/3(pqr)
  Constant/1 -> Rotor Assembly 1/4(Arm)
  [RotorA] -> Rotor Assembly 1/5(Tilt)
  Add/1 -> F/1
  Constant8/1 -> Rotor Assembly 1/6(TurnDirection)
  Rotor Assembly 1/1(F) -> [F1]
  Rotor Assembly 1/2(M) -> [M1]
  Rotor Assembly 2/1(F) -> [F2]
  In Bus Element2/1 -> Rotor Assembly 2/2(Vb)
  Constant3/1 -> Rotor Assembly 2/4(Arm)
  Constant5/1 -> Rotor Assembly 2/6(TurnDirection)
  In Bus Element3/1 -> Rotor Assembly 2/3(pqr)
  Rotor Assembly 2/2(M) -> [M2]
  Rotor Assembly 3/1(F) -> [F3]
  In Bus Element4/1 -> Rotor Assembly 3/2(Vb)
  Constant6/1 -> Rotor Assembly 3/4(Arm)
  Constant9/1 -> Rotor Assembly 3/6(TurnDirection)
  Constant7/1 -> Rotor Assembly 3/5(Tilt)
  In Bus Element5/1 -> Rotor Assembly 3/3(pqr)
  Rotor Assembly 3/2(M) -> [M3]
  Rotor Assembly 4/1(F) -> [F4]
  In Bus Element6/1 -> Rotor Assembly 4/2(Vb)
  Constant10/1 -> Rotor Assembly 4/4(Arm)
  Constant13/1 -> Rotor Assembly 4/6(TurnDirection)
  Constant11/1 -> Rotor Assembly 4/5(Tilt)
  In Bus Element7/1 -> Rotor Assembly 4/3(pqr)
  Rotor Assembly 4/2(M) -> [M4]
  [F1] -> Add/1
  [F2] -> Add/2
  [F3] -> Add/3
  [F4] -> Add/4
  [M4] -> Add1/4
  Add1/1 -> M/1
  [M3] -> Add1/3
  [M2] -> Add1/2
  [M1] -> Add1/1
  [w1] -> Bus Creator/1  "w1"
  [w2] -> Bus Creator/2  "w2"
  [w3] -> Bus Creator/3  "w3"
  [w4] -> Bus Creator/4  "w4"
  Bus Creator/1 -> RotorParameters/1
  [RotorA] -> Bus Creator/5  "Tilt1"
  [RotorB] -> Bus Creator/6  "Tilt2"
  Rotor Assembly 1/3(w) -> [w1]
  Rotor Assembly 2/3(w) -> [w2]
  Rho/1 -> [Rho]
  [RotorB] -> Rotor Assembly 2/5(Tilt)
  [Rho] -> Rotor Assembly 2/7(Rho)
  [Rho] -> Rotor Assembly 3/7(Rho)
  [Rho] -> Rotor Assembly 4/7(Rho)
  Rotor Assembly 3/3(w) -> [w3]
  Rotor Assembly 4/3(w) -> [w4]
  Sum/1 -> PID Controller/1
  Subsystem/1 -> Bus Selector/1, To Workspace/1
  Sum3/1 -> PID Controller3/1
  Sum2/1 -> PID Controller2/1
  Sum1/1 -> PID Controller1/1
  Bus Selector/1 -> Gain4/1  "<Mot_RPM_1>"
  Bus Selector/2 -> Gain5/1  "<Mot_RPM_2>"
  Bus Selector/3 -> Gain6/1  "<Mot_RPM_3>"
  Bus Selector/4 -> Gain7/1  "<Mot_RPM_4>"
  Gain/1 -> Gain12/1
  [Rho] -> Rotor Assembly 1/7(Rho)
  Bus Element In/1 -> Gain/1
  [Mot_RPM_SYS_1] -> Gain8/1
  Bus Element In3/1 -> Gain1/1
  [Mot_RPM_SYS_2] -> Gain9/1
  Bus Element In4/1 -> Gain2/1
  [Mot_RPM_SYS_3] -> Gain10/1
  Bus Element In5/1 -> Gain3/1
  [Mot_RPM_SYS_4] -> Gain11/1
  Gain4/1 -> Rotor Assembly 1/1(N)
  Gain6/1 -> Rotor Assembly 3/1(N)
  Gain7/1 -> Rotor Assembly 4/1(N)
  Gain1/1 -> Gain13/1
  Gain2/1 -> Gain14/1
  Gain3/1 -> Gain15/1
  Rate Transition/1 -> Sum/2
  Rate Transition1/1 -> Sum1/2
  Rate Transition2/1 -> Sum2/2
  Rate Transition3/1 -> Sum3/2
  Gain8/1 -> Rate Transition/1
  Gain9/1 -> Rate Transition1/1
  Gain10/1 -> Rate Transition2/1
  Gain11/1 -> Rate Transition3/1
  Gain12/1 -> Sum/1
  Gain13/1 -> Sum1/1
  Gain14/1 -> Sum2/1
  Gain15/1 -> Sum3/1
  PID Controller/1 -> Sum4/2
  Sum4/1 -> Subsystem/1
  PID Controller1/1 -> Sum5/2
  Sum5/1 -> Subsystem/2
  PID Controller2/1 -> Sum6/2
  Sum6/1 -> Subsystem/3
  PID Controller3/1 -> Sum7/2
  Sum7/1 -> Subsystem/4
  Tilt Servo Dynamics/1(Tilt1) -> [RotorA]
  Tilt Servo Dynamics/2(Tilt2) -> [RotorB]
  BusElementIn/1 -> Tilt Servo Dynamics/1(TiltA)
  BusElementIn1/1 -> Tilt Servo Dynamics/2(TiltB)
  BusElementIn2/1 -> Gain20/1
  BusElementIn3/1 -> Gain21/1
  BusElementIn4/1 -> Gain22/1
  BusElementIn5/1 -> Gain23/1
  Gain20/1 -> To Workspace7/1
  Gain21/1 -> To Workspace1/1
  Gain22/1 -> To Workspace8/1
  Gain23/1 -> To Workspace9/1
  Gain5/1 -> Rotor Assembly 2/1(N)
  [Mot_RPM_SYS_1] -> Rate Transition4/1
  Rate Transition4/1 -> To Workspace11/1
  Rate Transition5/1 -> To Workspace14/1
  [Mot_RPM_SYS_2] -> Rate Transition5/1
  Rate Transition6/1 -> To Workspace2/1
  Rate Transition7/1 -> To Workspace10/1
  [Mot_RPM_SYS_3] -> Rate Transition6/1
  [Mot_RPM_SYS_4] -> Rate Transition7/1
  [Drag_Torque1] -> Sum4/1
  [Drag_Torque2] -> Sum5/1
  [Drag_Torque3] -> Sum6/1
  [Drag_Torque4] -> Sum7/1
  [Drag_Torque1] -> Subsystem/5
  [Drag_Torque2] -> Subsystem/6
  [Drag_Torque3] -> Subsystem/7
  [Drag_Torque4] -> Subsystem/8
  [Mot_RPM_SYS_2] -> Rotor2 Drag Torque/1(Actuator)
  Rotor4 Drag Torque/1(Out1) -> [Drag_Torque4]
  Rotor3 Drag Torque/1(Out2) -> [Drag_Torque3]
  Rotor2 Drag Torque/1(Out2) -> [Drag_Torque2]
  Rotor1 Drag Torque/1(Out1) -> [Drag_Torque1]
  [Mot_RPM_SYS_1] -> Rotor1 Drag Torque/1(Actuator)
  [Mot_RPM_SYS_3] -> Rotor3 Drag Torque/1(Actuator)
  [Mot_RPM_SYS_4] -> Rotor4 Drag Torque/1(Actuator)
  [Drag_Torque4] -> To Workspace17/1
  [Drag_Torque3] -> To Workspace16/1
  [Drag_Torque2] -> To Workspace15/1
  [Drag_Torque1] -> To Workspace13/1

== system VTOLDynamics/Force and Moments/Weather Model ==
  AirData : Inport
  Xe : Inport  Port=2
  Euler : Inport  Port=3
  Simple Model : Subsystem  VariantControl=Wind==0
  Weather Model : Subsystem  VariantControl=Wind==1
  Wind_e : Outport
  Rho : Outport  Port=2

== system VTOLDynamics/Force and Moments/Aerodynamic Forces/Compute Air Data ==
  Vb : Inport  PortDimensions=3
  Rho : Inport  Port=2
  Bus Creator : BusCreator  Inputs=4
  Dynamic Pressure : aerolibasang/Dynamic Pressure
  "Incidence, Sideslip, & Airspeed" : aerolibasang/Incidence, Sideslip, & Airspeed
  Saturation : Saturate  Commented=on  UpperLimit=max(uavParams.aero.beta_latdir)  LowerLimit=min(uavParams.aero.beta_latdir)
  Saturation1 : Saturate  Commented=on  UpperLimit=max(uavParams.aero.alpha_lon)  LowerLimit=min(uavParams.aero.alpha_lon)
  AirData : Outport  VectorParamsAs1DForOutWhenUnconnected=off
  wires:
  Bus Creator/1 -> AirData/1
  "Incidence, Sideslip, & Airspeed"/1 -> Bus Creator/1  "alpha"
  Rho/1 -> Dynamic Pressure/2
  "Incidence, Sideslip, & Airspeed"/3 -> Bus Creator/3  "airspeed"
  Dynamic Pressure/1 -> Bus Creator/4  "q"
  Vb/1 -> "Incidence, Sideslip, & Airspeed"/1, Dynamic Pressure/1
  "Incidence, Sideslip, & Airspeed"/2 -> Bus Creator/2  "beta"

== system VTOLDynamics/Force and Moments/Aerodynamic Forces/Compute Body Frame Forces and Moments ==
  note: Dynamic pressure
  note: #5, 25/06/09, MH, Working
      | Check which coordinate system OpenVSPAero
      | uses, probability body coordinate system
      | Set CP as the origin of aero analysis
      | Set CG obtained from OpenVSP
  note: Velocity in body axes
  note: Aerodynamic coefficients
  note: Dynamic pressure can be computed by using vehicle's velocity and air density
  AirData : Inport
  CtrlSurfaces : Inport  Port=2
  Vb : Inport  Port=3
  p,q,r : Inport  Port=4
  Xe : Inport  Port=5
  "Aerodynamic Forces and Moments " : aerolibadyn/Aerodynamic Forces and Moments   inputAxes=Wind  outputForceAxes=Body  outputMomentAxes=Body  S=uavParams.geom.b*uavParams.geom.c  b=uavParams.geom.b  cbar=uavParams.geom.c
  Constant1 : Constant  Value=[0 0 0]
  Constant2 : Constant  Value=[0 0 0]
  Wind frame F& M : Subsystem
  Wind frame F& M_original : Subsystem  Commented=on
  F_b : Outport  Unit=kg*m/s^2  VectorParamsAs1DForOutWhenUnconnected=off
  M_b : Outport  Port=2  Unit=kg*m/s  VectorParamsAs1DForOutWhenUnconnected=off
  CtrlSurfacesStates : Outport  Port=3  Unit=kg*m/s  VectorParamsAs1DForOutWhenUnconnected=off
  wires:
  p,q,r/1 -> Wind frame F& M/3(p,q,r)
  "Aerodynamic Forces and Moments "/2 -> M_b/1
  "Aerodynamic Forces and Moments "/1 -> F_b/1
  CtrlSurfaces/1 -> Wind frame F& M/2(CtrlSurfaces)
  AirData/1 -> Wind frame F& M/1(Airdata)
  Vb/1 -> "Aerodynamic Forces and Moments "/5
  Constant1/1 -> "Aerodynamic Forces and Moments "/3
  Constant2/1 -> "Aerodynamic Forces and Moments "/4
  Wind frame F& M/2(coef) -> "Aerodynamic Forces and Moments "/1  "FM_W"
  Wind frame F& M/3(q) -> "Aerodynamic Forces and Moments "/2
  Wind frame F& M/1(CtrlSurfacesStates) -> CtrlSurfacesStates/1
  Xe/1 -> Wind frame F& M/4(Xe)

== system VTOLDynamics/Force and Moments/Ground Model/Friction Force ==
  V : Inport
  Fn : Inport  Port=2
  Product : Product
  Soft Coulomb Friction : Subsystem
  Unary Minus : UnaryMinus
  Friction : Outport
  wires:
  Unary Minus/1 -> Friction/1
  Fn/1 -> Product/2
  Soft Coulomb Friction/1(Out1) -> Product/1
  Product/1 -> Unary Minus/1
  V/1 -> Soft Coulomb Friction/1(V)

== system VTOLDynamics/Force and Moments/Ground Model/Normal Force ==
  Vz : Inport
  Z : Inport  Port=2
  Add : Sum
  Constant : Constant  Value=0  SampleTime=-1
  Damper : Gain  Gain=-sqrt(contact.spring*uavParams.geom.mass)
  Saturation : Saturate  UpperLimit=inf  LowerLimit=0  ZeroCross=off
  Spring Kp : Gain  Gain=-contact.spring
  Switch : Switch  Criteria=u2 > Threshold  SaturateOnIntegerOverflow=off  InputSameDT=off
  Unary Minus : UnaryMinus
  Unary Minus1 : UnaryMinus
  Normal : Outport
  wires:
  Add/1 -> Switch/3
  Constant/1 -> Switch/1
  Z/1 -> Unary Minus/1
  Switch/1 -> Saturation/1
  Damper/1 -> Add/2
  Spring Kp/1 -> Add/1
  Vz/1 -> Unary Minus1/1
  Saturation/1 -> Normal/1
  Unary Minus/1 -> Spring Kp/1, Switch/2
  Unary Minus1/1 -> Damper/1

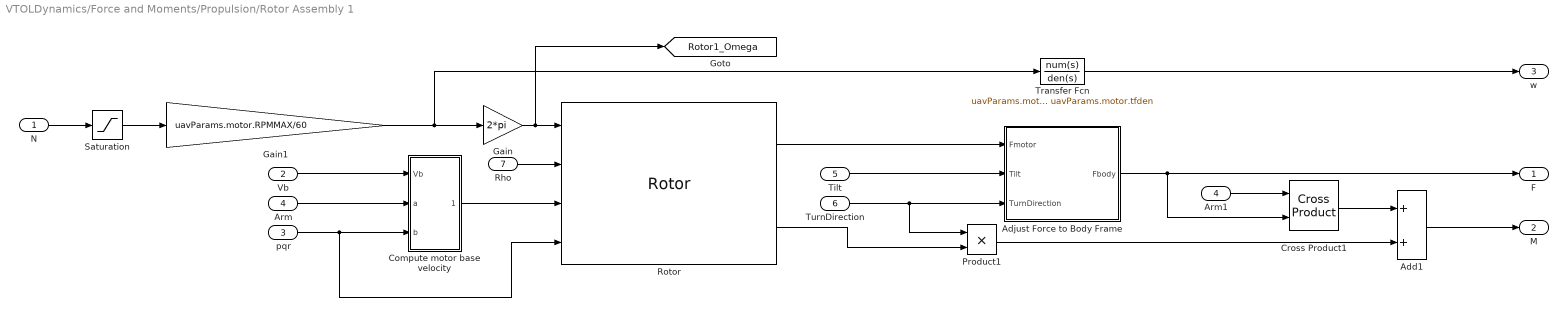
== system VTOLDynamics/Force and Moments/Propulsion/Rotor Assembly 1 ==
  N : Inport
  Vb : Inport  Port=2
  pqr : Inport  Port=3
  Arm : Inport  Port=4
  Tilt : Inport  Port=5
  TurnDirection : Inport  Port=6
  Rho : Inport  Port=7
  Add1 : Sum
  Adjust Force to Body Frame : Subsystem
  Arm1 : InportShadow  Port=4
  Compute motor base velocity : Subsystem
  Cross Product1 : matrix_library/Cross Product
  Gain : Gain  Gain=2*pi
  Gain1 : Gain  Gain=uavParams.motor.RPMMAX/60
  Product1 : Product
  Rotor : Rotor  modelMode=With flap effects  CT=uavParams.rotor.Ct  CQ=uavParams.rotor.Cq  Nb=uavParams.rotor.N  radius=uavParams.geom.PropDiameter/2  chord=uavParams.geom.PropChord  hingeOffset=uavParams.geom.PropOffHinge  clalpha=uavParams.geom.PropCLa  gamma=uavParams.geom.PropLock  thetaRoot=uavParams.geom.Propblroot  thetaTwist=uavParams.geom.Propbltwist
      settings: LibrarySourceBlock=aerolibrotor/Rotor
  Saturation : Saturate  UpperLimit=uavParams.motor.maxPWM  LowerLimit=uavParams.motor.minPWM
  Transfer Fcn : TransferFcn  Numerator=uavParams.motor.tfnum  Denominator=uavParams.motor.tfden
  F : Outport
  M : Outport  Port=2
  w : Outport  Port=3
  tag scope: Rotor1_Omega=global
  wires:
  TurnDirection/1 -> Adjust Force to Body Frame/3(TurnDirection), Product1/1
  Adjust Force to Body Frame/1(Fbody) -> F/1, Cross Product1/2
  Compute motor base velocity/1(Vmotor) -> Rotor/3
  Arm/1 -> Compute motor base velocity/2(a)
  Vb/1 -> Compute motor base velocity/1(Vb)
  Product1/1 -> Add1/2
  Cross Product1/1 -> Add1/1
  Arm1/1 -> Cross Product1/1
  Rho/1 -> Rotor/2
  Add1/1 -> M/1
  Rotor/2 -> Product1/2
  Gain/1 -> [Rotor1_Omega], Rotor/1
  pqr/1 -> Compute motor base velocity/3(b), Rotor/4
  Saturation/1 -> Gain1/1
  N/1 -> Saturation/1
  Gain1/1 -> Transfer Fcn/1, Gain/1
  Tilt/1 -> Adjust Force to Body Frame/2(Tilt)
  Rotor/1 -> Adjust Force to Body Frame/1(Fmotor)
  Transfer Fcn/1 -> w/1

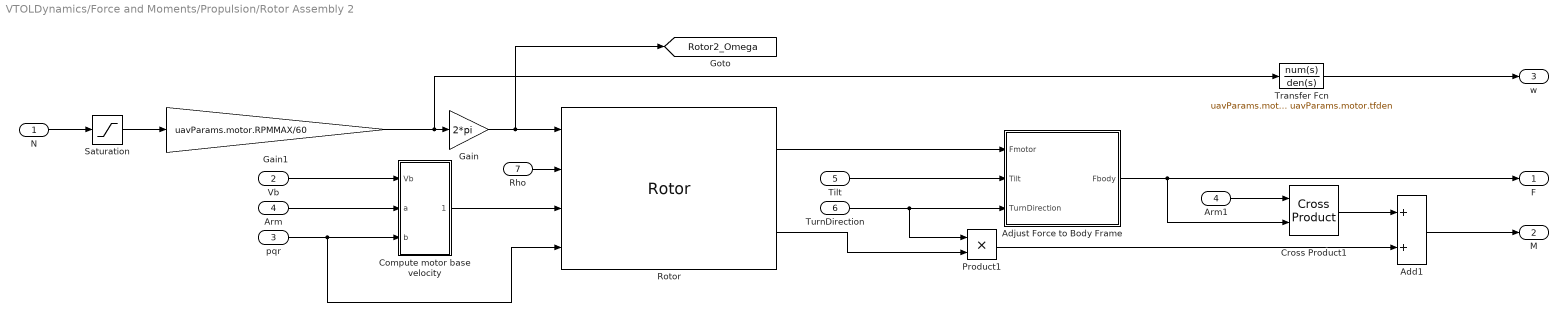
== system VTOLDynamics/Force and Moments/Propulsion/Rotor Assembly 2 ==
  N : Inport
  Vb : Inport  Port=2
  pqr : Inport  Port=3
  Arm : Inport  Port=4
  Tilt : Inport  Port=5
  TurnDirection : Inport  Port=6
  Rho : Inport  Port=7
  Add1 : Sum
  Adjust Force to Body Frame : Subsystem
  Arm1 : InportShadow  Port=4
  Compute motor base velocity : Subsystem
  Cross Product1 : matrix_library/Cross Product
  Gain : Gain  Gain=2*pi
  Gain1 : Gain  Gain=uavParams.motor.RPMMAX/60
  Product1 : Product
  Rotor : Rotor  modelMode=With flap effects  CT=uavParams.rotor.Ct  CQ=uavParams.rotor.Cq  Nb=uavParams.rotor.N  radius=uavParams.geom.PropDiameter/2  chord=uavParams.geom.PropChord  hingeOffset=uavParams.geom.PropOffHinge  clalpha=uavParams.geom.PropCLa  gamma=uavParams.geom.PropLock  thetaRoot=uavParams.geom.Propblroot  thetaTwist=uavParams.geom.Propbltwist
      settings: LibrarySourceBlock=aerolibrotor/Rotor
  Saturation : Saturate  UpperLimit=uavParams.motor.maxPWM  LowerLimit=uavParams.motor.minPWM
  Transfer Fcn : TransferFcn  Numerator=uavParams.motor.tfnum  Denominator=uavParams.motor.tfden
  F : Outport
  M : Outport  Port=2
  w : Outport  Port=3
  tag scope: Rotor2_Omega=global
  wires:
  TurnDirection/1 -> Adjust Force to Body Frame/3(TurnDirection), Product1/1
  Adjust Force to Body Frame/1(Fbody) -> F/1, Cross Product1/2
  Compute motor base velocity/1(Vmotor) -> Rotor/3
  Arm/1 -> Compute motor base velocity/2(a)
  Vb/1 -> Compute motor base velocity/1(Vb)
  Product1/1 -> Add1/2
  Cross Product1/1 -> Add1/1
  Arm1/1 -> Cross Product1/1
  Rho/1 -> Rotor/2
  Add1/1 -> M/1
  Rotor/2 -> Product1/2
  Gain/1 -> [Rotor2_Omega], Rotor/1
  pqr/1 -> Compute motor base velocity/3(b), Rotor/4
  Saturation/1 -> Gain1/1
  N/1 -> Saturation/1
  Gain1/1 -> Transfer Fcn/1, Gain/1
  Tilt/1 -> Adjust Force to Body Frame/2(Tilt)
  Rotor/1 -> Adjust Force to Body Frame/1(Fmotor)
  Transfer Fcn/1 -> w/1

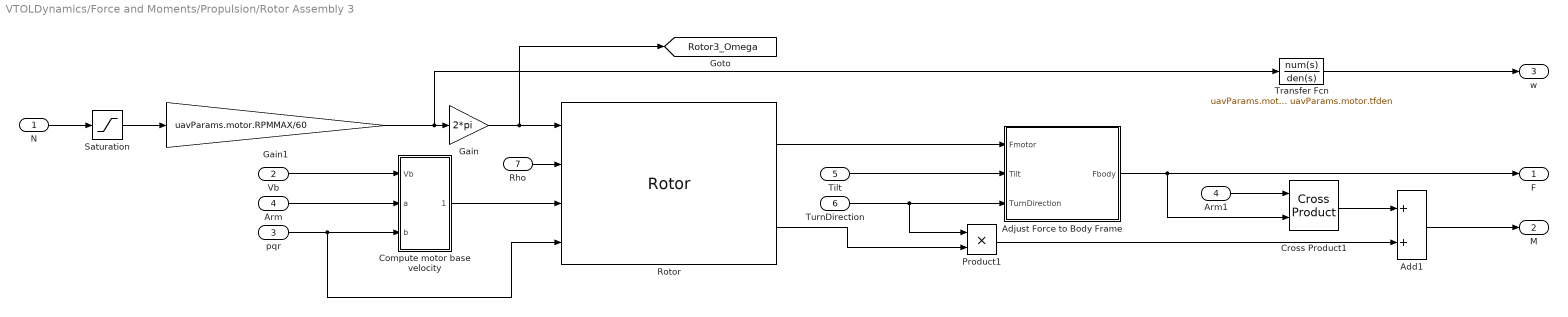
== system VTOLDynamics/Force and Moments/Propulsion/Rotor Assembly 3 ==
  N : Inport
  Vb : Inport  Port=2
  pqr : Inport  Port=3
  Arm : Inport  Port=4
  Tilt : Inport  Port=5
  TurnDirection : Inport  Port=6
  Rho : Inport  Port=7
  Add1 : Sum
  Adjust Force to Body Frame : Subsystem
  Arm1 : InportShadow  Port=4
  Compute motor base velocity : Subsystem
  Cross Product1 : matrix_library/Cross Product
  Gain : Gain  Gain=2*pi
  Gain1 : Gain  Gain=uavParams.motor.RPMMAX/60
  Product1 : Product
  Rotor : Rotor  modelMode=With flap effects  CT=uavParams.rotor.Ct  CQ=uavParams.rotor.Cq  Nb=uavParams.rotor.N  radius=uavParams.geom.PropDiameter/2  chord=uavParams.geom.PropChord  hingeOffset=uavParams.geom.PropOffHinge  clalpha=uavParams.geom.PropCLa  gamma=uavParams.geom.PropLock  thetaRoot=uavParams.geom.Propblroot  thetaTwist=uavParams.geom.Propbltwist
      settings: LibrarySourceBlock=aerolibrotor/Rotor
  Saturation : Saturate  UpperLimit=uavParams.motor.maxPWM  LowerLimit=uavParams.motor.minPWM
  Transfer Fcn : TransferFcn  Numerator=uavParams.motor.tfnum  Denominator=uavParams.motor.tfden
  F : Outport
  M : Outport  Port=2
  w : Outport  Port=3
  tag scope: Rotor3_Omega=global
  wires:
  TurnDirection/1 -> Adjust Force to Body Frame/3(TurnDirection), Product1/1
  Adjust Force to Body Frame/1(Fbody) -> F/1, Cross Product1/2
  Compute motor base velocity/1(Vmotor) -> Rotor/3
  Arm/1 -> Compute motor base velocity/2(a)
  Vb/1 -> Compute motor base velocity/1(Vb)
  Product1/1 -> Add1/2
  Cross Product1/1 -> Add1/1
  Arm1/1 -> Cross Product1/1
  Rho/1 -> Rotor/2
  Add1/1 -> M/1
  Rotor/2 -> Product1/2
  Gain/1 -> [Rotor3_Omega], Rotor/1
  pqr/1 -> Compute motor base velocity/3(b), Rotor/4
  Saturation/1 -> Gain1/1
  N/1 -> Saturation/1
  Gain1/1 -> Transfer Fcn/1, Gain/1
  Tilt/1 -> Adjust Force to Body Frame/2(Tilt)
  Rotor/1 -> Adjust Force to Body Frame/1(Fmotor)
  Transfer Fcn/1 -> w/1

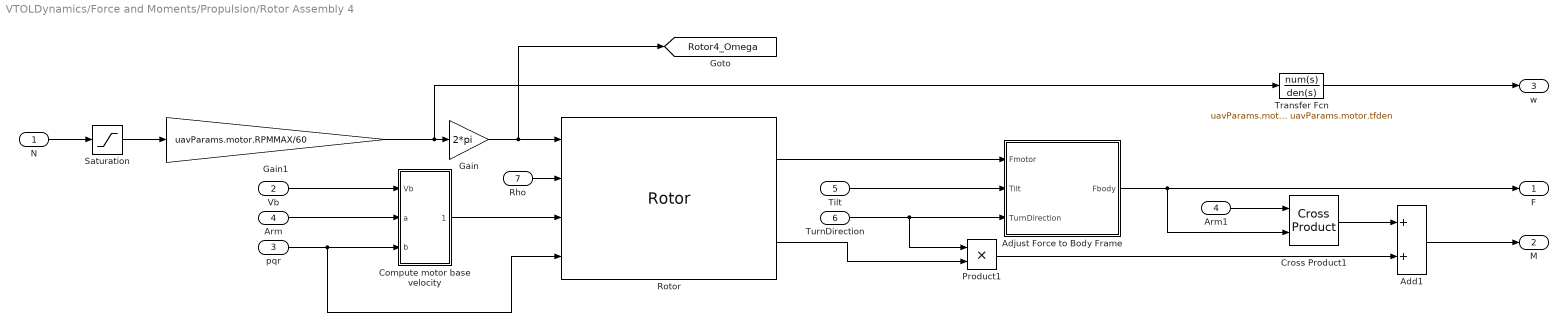
== system VTOLDynamics/Force and Moments/Propulsion/Rotor Assembly 4 ==
  N : Inport
  Vb : Inport  Port=2
  pqr : Inport  Port=3
  Arm : Inport  Port=4
  Tilt : Inport  Port=5
  TurnDirection : Inport  Port=6
  Rho : Inport  Port=7
  Add1 : Sum
  Adjust Force to Body Frame : Subsystem
  Arm1 : InportShadow  Port=4
  Compute motor base velocity : Subsystem
  Cross Product1 : matrix_library/Cross Product
  Gain : Gain  Gain=2*pi
  Gain1 : Gain  Gain=uavParams.motor.RPMMAX/60
  Product1 : Product
  Rotor : Rotor  modelMode=With flap effects  CT=uavParams.rotor.Ct  CQ=uavParams.rotor.Cq  Nb=uavParams.rotor.N  radius=uavParams.geom.PropDiameter/2  chord=uavParams.geom.PropChord  hingeOffset=uavParams.geom.PropOffHinge  clalpha=uavParams.geom.PropCLa  gamma=uavParams.geom.PropLock  thetaRoot=uavParams.geom.Propblroot  thetaTwist=uavParams.geom.Propbltwist
      settings: LibrarySourceBlock=aerolibrotor/Rotor
  Saturation : Saturate  UpperLimit=uavParams.motor.maxPWM  LowerLimit=uavParams.motor.minPWM
  Transfer Fcn : TransferFcn  Numerator=uavParams.motor.tfnum  Denominator=uavParams.motor.tfden
  F : Outport
  M : Outport  Port=2
  w : Outport  Port=3
  tag scope: Rotor4_Omega=global
  wires:
  TurnDirection/1 -> Adjust Force to Body Frame/3(TurnDirection), Product1/1
  Adjust Force to Body Frame/1(Fbody) -> F/1, Cross Product1/2
  Compute motor base velocity/1(Vmotor) -> Rotor/3
  Arm/1 -> Compute motor base velocity/2(a)
  Vb/1 -> Compute motor base velocity/1(Vb)
  Product1/1 -> Add1/2
  Cross Product1/1 -> Add1/1
  Arm1/1 -> Cross Product1/1
  Rho/1 -> Rotor/2
  Add1/1 -> M/1
  Rotor/2 -> Product1/2
  Gain/1 -> [Rotor4_Omega], Rotor/1
  pqr/1 -> Compute motor base velocity/3(b), Rotor/4
  Saturation/1 -> Gain1/1
  N/1 -> Saturation/1
  Gain1/1 -> Transfer Fcn/1, Gain/1
  Tilt/1 -> Adjust Force to Body Frame/2(Tilt)
  Rotor/1 -> Adjust Force to Body Frame/1(Fmotor)
  Transfer Fcn/1 -> w/1
